simulink model "g1_G1234_p_sim"  (R2025b)
settings: Solver=VariableStepAuto  StartTime=0.0  StopTime=3  MaxStep=50e-6  RelTol=1e-3
values from neighbouring files (symbols this model uses):
  K234 = 102.9 / K0    (= 51.45)    [g1_ini_01.m]
  T23 = (t23_10/a2_10 + t23_50/a2_50 + t23_90/a2_90) / 3    [g1_ini_01.m]
  Tt = t1 - t0    (= 0.0025)    [g1_ini_01.m]
settings Model: Creator=PMIC  LastModifiedBy=andre
settings DataIOCC: SaveOutput=off  SignalLogging=off  DSMLogging=off  SaveTime=off  ReturnWorkspaceOutputs=off
settings RTWCC: GPUComputeCapability=3.5

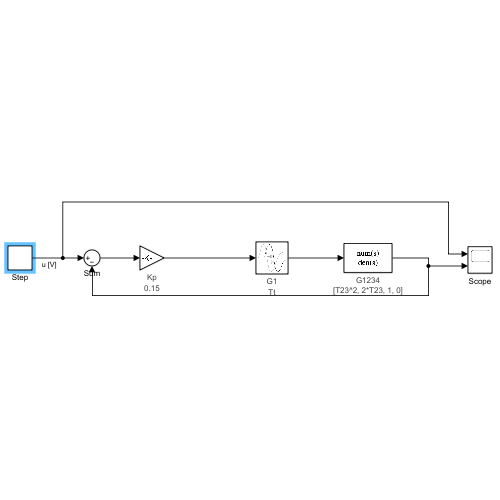
[thumbnail: Simulink's stored preview of the top-level diagram]
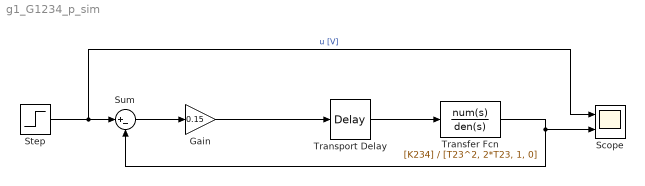
== system g1_G1234_p_sim ==
  Gain : Gain  Description=Kp  Gain=0.15
      settings: AttributesFormatString=|
      | %<Description>
      | %<Gain>
  Scope : Scope  NumInputPorts=2
      settings: ActiveDisplayYMinimum=-0.61062673994946515  ActiveDisplayYMaximum=2.629264223605364
  Step : Step  Time=0.05  After=0  SampleTime=0
  Sum : Sum  Inputs=|+-
  Transfer Fcn : TransferFcn  Description=G1234  Numerator=[K234]  Denominator=[T23^2, 2*T23, 1, 0]
      settings: AttributesFormatString=|
      | %<Description>
      | %<Denominator>
  Transport Delay : TransportDelay  Description=G1  DelayTime=Tt
      settings: AttributesFormatString=|
      | %<Description>
      | %<DelayTime>
  wires:
  Step/1 -> Scope/1, Sum/1  "u [V]"
  Transport Delay/1 -> Transfer Fcn/1
  Transfer Fcn/1 -> Sum/2, Scope/2
  Sum/1 -> Gain/1
  Gain/1 -> Transport Delay/1
